simulink model "MPU_6050_example"  (R2019b)
settings: Solver=FixedStepDiscrete  StartTime=0.0  StopTime=5  FixedStep=0.001  RelTol=1e-3  EnableMultiTasking=on
settings Model: SimulationMode=external  SILPILModeSetting=veronly  ExtModeTrigDuration=2  Creator=ganna  LastModifiedBy=ganna
settings DataIOCC: ReturnWorkspaceOutputs=off
settings OptimizationCC: EnhancedBackFolding=on  PassReuseOutputArgsAs=Individual arguments  ZeroExternalMemoryAtStartup=off  ZeroInternalMemoryAtStartup=off  MaxStackSize=64  OptimizeBlockOrder=speed  DifferentSizesBufferReuse=on  OptimizationCustomize=off  EfficientTunableParamExpr=on
settings DebuggingCC: ParameterTunabilityLossMsg=error
settings HardwareCC: ProdBitPerInt=16  ProdBitPerPointer=16  ProdBitPerSizeT=16  ProdBitPerPtrDiffT=16  ProdLargestAtomicFloat=None  ProdWordSize=8  ProdHWDeviceType=Atmel->AVR  UseEmbeddedCoderFeatures=off
settings SFSimCC: MATLABDynamicMemAlloc=off
settings RTWCC: SystemTargetFile=ert.tlc  HardwareBoard=Arduino Mega 2560  TLCOptions=-aInlineSetEventsForThisBaseRateFcn=TLC_FALSE -aSuppressMultiTaskScheduler=TLC_FALSE -aRateBasedStepFcn=1  TemplateMakefile=ert_default_tmf  GenerateReport=on  Toolchain=Arduino AVR  BuildConfiguration=Faster Runs  IncludeHyperlinkInReport=on  LaunchReport=on  GenerateTraceInfo=on  GenerateTraceReport=on  GenerateTraceReportSl=on  GenerateTraceReportSf=on  GenerateTraceReportEml=on
settings CodeAppCC: ForceParamTrailComments=on  IgnoreCustomStorageClasses=off  OperatorAnnotations=on  SimulinkDataObjDesc=on  SFDataObjDesc=on  InsertBlockDesc=on
settings ERTTargetCC: SupportContinuousTime=on  SupportNonInlinedSFcns=on  SupportVariableSizeSignals=on  ExtModeStaticAllocSize=2048

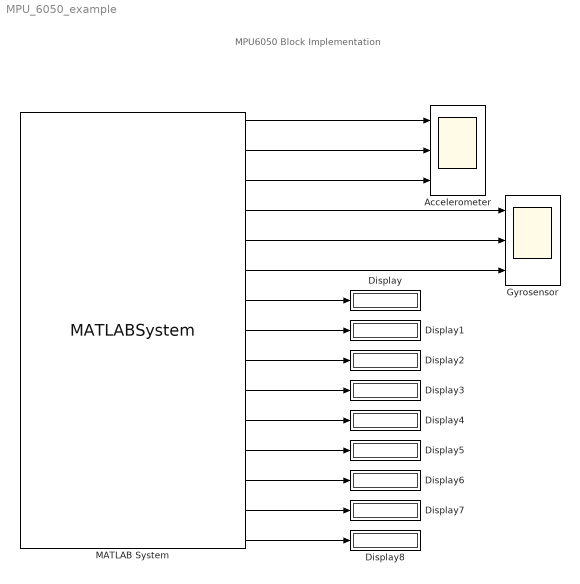
== system MPU_6050_example ==
  note: MPU6050 Block Implementation
  Accelerometer : Scope  NumInputPorts=3
  Display{,1..8} (9 alike) : Display
  Gyrosensor : Scope  NumInputPorts=3
  MATLAB System : MATLABSystem  System=MPU6050
      mask Type: MPU6050
      mask Display:
      | image('MPU6050.png');
      | port_label('output',1,'acc_x');
      | port_label('output',2,'acc_y');
      | port_label('output',3,'acc_z');
      | port_label('output',4,'gyro_x');
      | port_label('output',5,'gyro_y');
      | port_label('output',6,'gyro_z');
      | port_label('output',7,'acc_angl_x');
      | port_label('output',8,'acc_angl_y');
      | port_label('output',9,'gyro_angl_x');
      | port_label('output',10,'gyro_angl_y');
      | port_label('output',11,'gyro_angl_z');
      | port_label('output',12,'angl_x');
      | port_label('output',13,'angl_y');
      | port_label('output',14,'angl_z');
      | port_label('output',15,'temp');
  wires:
  MATLAB System/1 -> Accelerometer/1
  MATLAB System/2 -> Accelerometer/2
  MATLAB System/3 -> Accelerometer/3
  MATLAB System/4 -> Gyrosensor/1
  MATLAB System/5 -> Gyrosensor/2
  MATLAB System/6 -> Gyrosensor/3
  MATLAB System/7 -> Display/1
  MATLAB System/8 -> Display1/1
  MATLAB System/9 -> Display2/1
  MATLAB System/11 -> Display4/1
  MATLAB System/10 -> Display3/1
  MATLAB System/12 -> Display5/1
  MATLAB System/13 -> Display6/1
  MATLAB System/14 -> Display7/1
  MATLAB System/15 -> Display8/1
